simulink model "Part_B_DSB_LC_Modulation"  (R2023a)
settings: Solver=VariableStepAuto  StartTime=0.0  StopTime=1  RelTol=1e-3
values from neighbouring files (symbols this model uses):
  Fs = 1000    [Part_A_DSB_LC_Modulation.m]
settings Model: Creator=dscmu  LastModifiedBy=dscmu
settings OptimizationCC: ReuseModelBlockBuffer=off

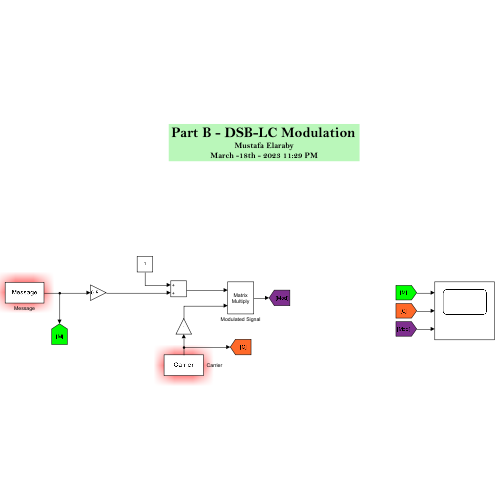
[thumbnail: Simulink's stored preview of the top-level diagram]
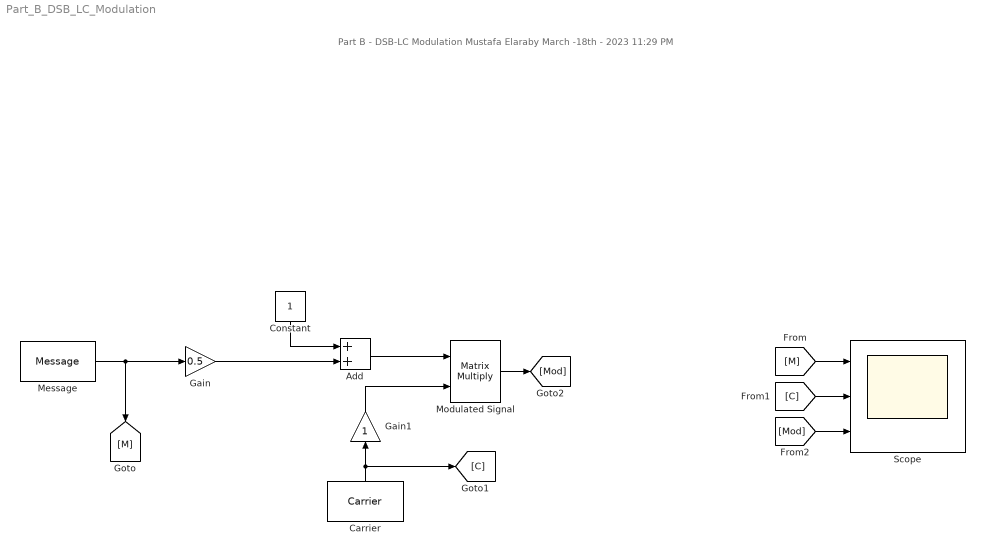
== system Part_B_DSB_LC_Modulation ==
  note: Part B - DSB-LC Modulation
      | Mustafa Elaraby
      | March -18th - 2023 11:29 PM
  Add : Sum
  Carrier : FromWorkspace  VariableName=Carrier  SampleTime=1/Fs  OutputAfterFinalValue=Holding final value
  Constant : Constant
  Gain : Gain  Gain=0.5
  Gain1 : Gain
  Message : FromWorkspace  VariableName=Message  SampleTime=1/Fs
  Modulated Signal : Product  Multiplication=Matrix(*)
  Scope : Scope  NumInputPorts=3
  wires:
  Gain/1 -> Add/2
  Constant/1 -> Add/1
  Add/1 -> Modulated Signal/1
  Message/1 -> [M], Gain/1
  Carrier/1 -> [C], Gain1/1
  Modulated Signal/1 -> [Mod]
  [Mod] -> Scope/3
  [C] -> Scope/2
  [M] -> Scope/1
  Gain1/1 -> Modulated Signal/2
